simulink model "Engine_MvMdl_Ptbs_V1_slprjref"  (R2018b)
settings: Solver=VariableStepAuto  StartTime=0.0  StopTime=660  FixedStep=0.001  EnableMultiTasking=on
PreLoadFcn:
  | Engine_MapMdl_Ptbs_V1_BusInfo
model workspace (MAT data in the model file):
  DiffRatio = 3.421
  EV_current = 200
  EV_motion = [20 4 0.8]
  EV_sf = 2000
  EngDriveRatio = 0.813008130081
  Fs = 0
  Fv = 0.0025
  Jcomp = 0.0227
  Jengine = 0.22
  Ki = 251.3274
  Kisa = 346.6583
  Kp_d = 0.47149
  Kp_q = 0.52125
  Ksa = 85.4316
  Ksf = 1996.2651
  Ld = 0.0003752
  Ldq = [0.0003752 0.0004148]
  Lq = 0.0004148
  Mechanical = [0.0227 0.0025 0]
  MotGbRatio = 1
  P = 4
  PolePairs = 4
  RWheel = 0.3
  Rs = 0.2
  T_max = 120
  T_mtpa = [0 13.3131834767 26.6278836885 39.9456159322 53.2678926341 66.5962219318 79.9321062746 93.277041051 106.632513247 120.000000141]
  MCOS : class17 (value not decoded)
  MCOS : class17 (value not decoded)
  ba = 3.4029
  id_mtpa = [0 -0.114523352646 -0.457989076459 -1.03008464374 -1.83029075221 -2.85788367342 -4.11193850568 -5.59133329791 -7.29475400168 -9.22070020138]
  idq0 = [0 0]
  idq_limits = [-9.220699542 166.993501392 167.247872355]
  iq_mtpa = [0 18.5827440345 37.1633719111 55.7397734896 74.3098506185 92.871523015 111.422734008 129.961456105 148.485696337 166.993501356]
  MCOS : class17 (value not decoded)
  MCOS : class17 (value not decoded)
  lambda_pm = 0.1194
  mechanical = [0.0227 0.0025 0]
  mot : struct (value not decoded)
  omega_init = 0
  theta_init = 0
  MCOS : class17 (value not decoded)
libraries: autolibsharedmappedengines x1
(part 3 of 3)

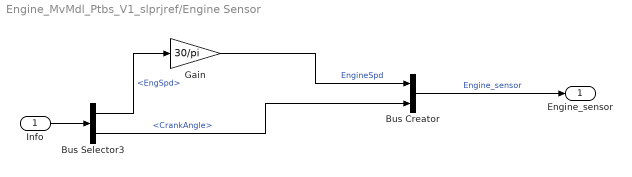
== system Engine_MvMdl_Ptbs_V1_slprjref/Engine Sensor ==
  Info : Inport
  Bus Creator : BusCreator  Inputs=2  OutDataTypeStr=Bus: Engine_sensor_Bus
      settings: AttributesFormatString=%<OutDataTypeStr>
  Bus Selector3 : BusSelector  OutputSignals=EngSpd,CrankAngle
  Gain : Gain  Gain=30/pi
  Engine_sensor : Outport
  wires:
  Gain/1 -> Bus Creator/1  "EngineSpd"
  Bus Creator/1 -> Engine_sensor/1  "Engine_sensor"
  Info/1 -> Bus Selector3/1
  Bus Selector3/2 -> Bus Creator/2  "<CrankAngle>"
  Bus Selector3/1 -> Gain/1  "<EngSpd>"

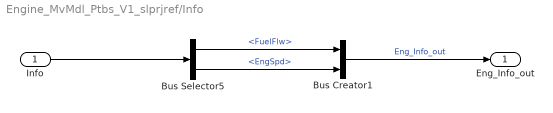
== system Engine_MvMdl_Ptbs_V1_slprjref/Info ==
  Info : Inport
  Bus Creator1 : BusCreator  Inputs=2  OutDataTypeStr=Bus: Eng_Info_out_Bus
      settings: AttributesFormatString=%<OutDataTypeStr>
  Bus Selector5 : BusSelector  OutputSignals=FuelFlw,EngSpd
  Eng_Info_out : Outport
  wires:
  Bus Creator1/1 -> Eng_Info_out/1  "Eng_Info_out"
  Info/1 -> Bus Selector5/1
  Bus Selector5/2 -> Bus Creator1/2  "<EngSpd>"
  Bus Selector5/1 -> Bus Creator1/1  "<FuelFlw>"
